simulink model "Control_Schematic_9"  (Simulink 8.3)
settings: Solver=FixedStepDiscrete  StartTime=0.0  StopTime=100  FixedStep=Ts  RelTol=1e-3
values from neighbouring files (symbols this model uses):
  b = 156    [StartUp_1.m]    (also in StartUp_11_Validation.m; StartUp_3.m; StartUp_4.m; StartUp_7.m)
  Eps = .1    (= 0.1)    [StartUp_9.m]
  K1 = PolyCon(1,2)    [StartUp_1.m]    (also in StartUp_4.m = 1; StartUp_7.m = 16; StartUp_8.m = 16; StartUp_9.m = 0.23)
  k2 = floor(rk(2,1))    [StartUp_9.m]
  K2 = 2    [StartUp_4.m]    (also in StartUp_7.m = 8; StartUp_8.m = 8; StartUp_9.m = 0.83)
  k3 = kk    [StartUp_9.m]
  K3 = 12000    [StartUp_9.m]
  ka = .5    (= 0.5)    [StartUp_9.m]
  Kn = .0019    (= 0.0019)    [StartUp_9.m]
  R = 50    [StartUp_1.m]    (also in StartUp_3.m; StartUp_4.m; StartUp_7.m; StartUp_8.m)
  Ts = 1/1000    (= 0.001)    [StartUp_1.m]    (also in StartUp_11_Validation.m = 0.01; StartUp_3.m; StartUp_4.m; StartUp_7.m)
  x_0 = 2500    [StartUp_9.m]
  y_0 = 2500    [StartUp_9.m]
undefined symbols (not defined in the file or in its folder): DiscIntNeverNeededParam
undefined symbols (not defined in the file): ADAMS_cwd, ADAMS_exec, ADAMS_host, ADAMS_init, ADAMS_inputs, ADAMS_outputs, ADAMS_prefix, ADAMS_static, ADAMS_sysdir
libraries: dspinverses x1, simulink x1
settings Model: Creator=baqumau  LastModifiedBy=baqumau
settings DataIOCC: SignalLoggingSaveFormat=Dataset
settings DebuggingCC: UnderspecifiedInitializationDetection=Simplified  StateNameClashWarn=none
settings GRTTargetCC: CombineOutputUpdateFcns=on  GRTInterface=off

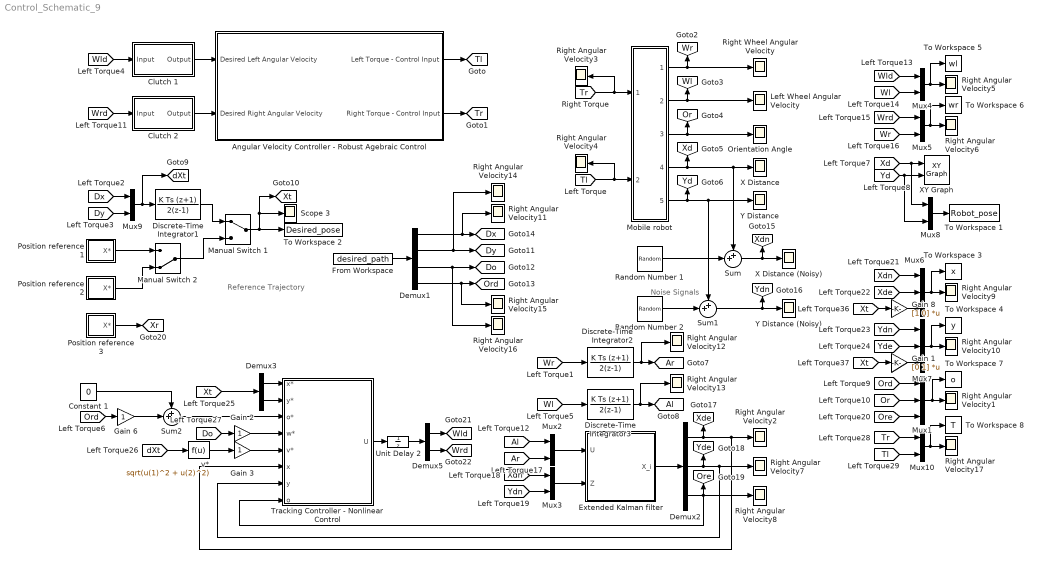
== system Control_Schematic_9 ==
  note: Noise Signals
  note: Reference Trajectory
  Angular Velocity Controller - Robust Agebraic Control : Subsystem
  Clutch 1 : Subsystem
  Clutch 2 : Subsystem
  Constant 1 : Constant  Value=0
  Demux1 : Demux
  Demux2 : Demux  Outputs=3
  Demux3 : Demux  Outputs=2
  Demux5 : Demux  Outputs=2
  Discrete-Time Integrator1 : DiscreteIntegrator  IntegratorMethod=Integration: Trapezoidal  gainval=1  InitialCondition=[x_0,y_0]'  SampleTime=Ts  ICPrevOutput=DiscIntNeverNeededParam  ICPrevScaledInput=DiscIntNeverNeededParam
  Discrete-Time Integrator2 : DiscreteIntegrator  IntegratorMethod=Integration: Trapezoidal  gainval=1  SampleTime=Ts  ICPrevOutput=DiscIntNeverNeededParam  ICPrevScaledInput=DiscIntNeverNeededParam
  Discrete-Time Integrator3 : DiscreteIntegrator  IntegratorMethod=Integration: Trapezoidal  gainval=1  SampleTime=Ts  ICPrevOutput=DiscIntNeverNeededParam  ICPrevScaledInput=DiscIntNeverNeededParam
  Extended Kalman filter : Subsystem
  From Workspace : FromWorkspace  VariableName=desired_path  SampleTime=Ts  OutputAfterFinalValue=Holding final value
  Gain 1 : Gain  Gain=[0 1]  Multiplication=Matrix(K*u)
  Gain 2 : Gain
  Gain 3 : Gain
  Gain 6 : Gain
  Gain 8 : Gain  Gain=[1 0]  Multiplication=Matrix(K*u)
  Left Wheel Angular Velocity : Scope
      settings: YMin=-1  YMax=1  SaveName=ScopeData2
  Manual Switch 1 : ManualSwitch
  Manual Switch 2 : ManualSwitch  CurrentSetting=0
  Mobile robot : Subsystem
  Mux1 : Mux  Inputs=3
  Mux{2..5,8..10} (7 alike) : Mux  Inputs=2
  Mux6 : Mux  Inputs=3
  Mux7 : Mux  Inputs=3
  Orientation Angle : Scope
      settings: YMin=-4  YMax=4
  Position reference 1 : Subsystem
  Position reference 2 : Subsystem
  Position reference 3 : Subsystem
  Random Number 1 : RandomNumber  Variance=.5  Seed=6
  Random Number 2 : RandomNumber  Variance=.5  Seed=8
  Right Angular Velocity{1..17} (17 alike) : Scope
      Right Angular Velocity1 settings: SaveName=ScopeData27
      Right Angular Velocity10 settings: YMin=0  YMax=5000  SaveName=ScopeData36
      Right Angular Velocity11 settings: YMin=0  YMax=4500  SaveName=ScopeData11
      Right Angular Velocity12 settings: YMin=-3  YMax=30  SaveName=ScopeData39
      Right Angular Velocity13 settings: YMin=-3  YMax=3  SaveName=ScopeData40
      Right Angular Velocity14 settings: TimeRange=500  YMin=0  YMax=4500  SaveName=ScopeData13
      Right Angular Velocity15 settings: YMin=-3.141592653589793  YMax=3.141592653589793  SaveName=ScopeData15
      Right Angular Velocity16 settings: YMin=0  YMax=4500  SaveName=ScopeData16
      Right Angular Velocity17 settings: YMax=25  SaveName=ScopeData5
      Right Angular Velocity2 settings: YMin=2400  YMax=2600  SaveName=ScopeData24
      Right Angular Velocity3 settings: YMin=-25  YMax=25  SaveName=ScopeData7
      Right Angular Velocity4 settings: YMin=-25  YMax=25  SaveName=ScopeData8
      Right Angular Velocity5 settings: YMax=25  SaveName=ScopeData9
      Right Angular Velocity6 settings: TimeRange=388.54  YMin=-3  YMax=25  SaveName=ScopeData10
      Right Angular Velocity7 settings: YMin=0  YMax=5000  SaveName=ScopeData25
      Right Angular Velocity8 settings: YMin=-3.141592653589793  YMax=3.141592653589793  SaveName=ScopeData26
      Right Angular Velocity9 settings: YMin=0  YMax=5000  SaveName=ScopeData35
  Right Wheel Angular Velocity : Scope
      settings: YMin=-1  YMax=1  SaveName=ScopeData3
  Scope 3 : Scope
      settings: YMin=100  YMax=5000  SaveName=ScopeData37
  Sum : Sum  Inputs=++|
  Sum1 : Sum  Inputs=++|
  Sum2 : Sum  Inputs=++|
  To Workspace 1 : ToWorkspace  VariableName=Robot_pose  SaveFormat=Structure With Time  SampleTime=-1
  To Workspace 2 : ToWorkspace  VariableName=Desired_pose  SaveFormat=Structure With Time  SampleTime=-1
  To Workspace 3 : ToWorkspace  VariableName=x  SaveFormat=Structure With Time  SampleTime=-1
  To Workspace 4 : ToWorkspace  VariableName=y  SaveFormat=Structure With Time  SampleTime=-1
  To Workspace 5 : ToWorkspace  VariableName=wl  SaveFormat=Structure With Time  SampleTime=-1
  To Workspace 6 : ToWorkspace  VariableName=wr  SaveFormat=Structure With Time  SampleTime=-1
  To Workspace 7 : ToWorkspace  VariableName=o  SaveFormat=Structure With Time  SampleTime=-1
  To Workspace 8 : ToWorkspace  VariableName=T  SaveFormat=Structure With Time  SampleTime=-1
  Tracking Controller - Nonlinear Control : Subsystem
  Unit Delay 2 : UnitDelay  SampleTime=-1
  X Distance : Scope
      settings: YMin=0  YMax=5000  SaveName=ScopeData4
  X Distance (Noisy) : Scope
      settings: YMin=0  YMax=2600  SaveName=ScopeData19
  XY Graph : simulink/Sinks/XY Graph  xmin=0  xmax=5000  ymin=0  ymax=5000  st=Ts
  Y Distance : Scope
      settings: YMin=0  YMax=5000
  Y Distance (Noisy) : Scope
      settings: YMin=0  YMax=2600  SaveName=ScopeData21
  v* : Fcn  Expr=sqrt(u(1)^2 + u(2)^2)
  tag scope: Al=global, Ar=global, Do=global, Dx=global, Dy=global, Or=global, Ord=global, Ore=global, Tl=global, Tr=global, Wl=global, Wld=global, Wr=global, Wrd=global, Xd=global, Xde=global, Xdn=global, Xr=global, Xt=global, Yd=global, Yde=global, Ydn=global, dXt=global
  wires:
  Mobile robot/1(Wrw) -> Right Wheel Angular Velocity/1, [Wr]
  Mobile robot/2(Wlw) -> Left Wheel Angular Velocity/1, [Wl]
  Mobile robot/3(Alpha) -> Orientation Angle/1, [Or]
  Mobile robot/4(X_Dist) -> Sum/1, X Distance/1, [Xd]
  Mobile robot/5(Y_Dist) -> Y Distance/1, Sum1/1, [Yd]
  [Tr] -> Mobile robot/1(Trw), Right Angular Velocity3/1
  [Tl] -> Mobile robot/2(Tlw), Right Angular Velocity4/1
  [Wld] -> Mux4/1
  [Wl] -> Mux4/2
  Mux4/1 -> To Workspace 5/1, Right Angular Velocity5/1
  [Wrd] -> Mux5/1
  [Wr] -> Mux5/2
  Mux5/1 -> To Workspace 6/1, Right Angular Velocity6/1
  [Xd] -> Mux8/1, XY Graph/1
  [Yd] -> Mux8/2, XY Graph/2
  [Ord] -> Mux1/1
  [Or] -> Mux1/2
  Mux1/1 -> To Workspace 7/1, Right Angular Velocity1/1
  Random Number 1/1 -> Sum/2
  Sum1/1 -> Y Distance (Noisy)/1, [Ydn]
  Sum/1 -> [Xdn], X Distance (Noisy)/1
  [Ar] -> Mux2/2
  [Al] -> Mux2/1
  [Ydn] -> Mux3/2
  [Xdn] -> Mux3/1
  Mux2/1 -> Extended Kalman filter/1(U)
  Mux3/1 -> Extended Kalman filter/2(Z)
  Demux2/2 -> [Yde], Tracking Controller - Nonlinear Control/7(y), Right Angular Velocity7/1
  Demux2/3 -> Tracking Controller - Nonlinear Control/8(o), [Ore], Right Angular Velocity8/1
  Demux2/1 -> [Xde], Tracking Controller - Nonlinear Control/6(x), Right Angular Velocity2/1
  [Ore] -> Mux1/3
  [Xdn] -> Mux6/1
  Mux6/1 -> To Workspace 3/1, Right Angular Velocity9/1
  [Xde] -> Mux6/2
  [Ydn] -> Mux7/1
  Mux7/1 -> To Workspace 4/1, Right Angular Velocity10/1
  [Yde] -> Mux7/2
  Mux8/1 -> To Workspace 1/1
  [Xt] -> Gain 8/1
  Gain 8/1 -> Mux6/3
  [Xt] -> Gain 1/1
  Gain 1/1 -> Mux7/3
  Manual Switch 1/1 -> [Xt], Scope 3/1, To Workspace 2/1
  Demux1/1 -> Right Angular Velocity11/1, [Dx]
  Demux1/2 -> Right Angular Velocity14/1, [Dy]
  Demux1/3 -> Right Angular Velocity16/1, [Do]
  Demux1/4 -> Right Angular Velocity15/1, [Ord]
  From Workspace/1 -> Demux1/1
  [Dx] -> Mux9/1
  [Dy] -> Mux9/2
  Mux9/1 -> [dXt], Discrete-Time Integrator1/1
  Discrete-Time Integrator1/1 -> Manual Switch 1/1
  Position reference 1/1(X*) -> Manual Switch 2/1
  Manual Switch 2/1 -> Manual Switch 1/2
  Position reference 2/1(X*) -> Manual Switch 2/2
  Position reference 3/1(X*) -> [Xr]
  Demux5/2 -> [Wrd]
  Demux5/1 -> [Wld]
  Discrete-Time Integrator2/1 -> Right Angular Velocity12/1, [Ar]
  [Wr] -> Discrete-Time Integrator2/1
  Discrete-Time Integrator3/1 -> Right Angular Velocity13/1, [Al]
  [Wl] -> Discrete-Time Integrator3/1
  Tracking Controller - Nonlinear Control/1(U) -> Unit Delay 2/1
  Demux3/1 -> Tracking Controller - Nonlinear Control/1(x*)
  Demux3/2 -> Tracking Controller - Nonlinear Control/2(y*)
  [Xt] -> Demux3/1
  [Wld] -> Clutch 1/1(Input)
  [Wrd] -> Clutch 2/1(Input)
  [Do] -> Gain 2/1
  v*/1 -> Gain 3/1
  [dXt] -> v*/1
  Clutch 1/1(Output) -> Angular Velocity Controller - Robust Agebraic Control/1(Desired Left Angular Velocity)
  Clutch 2/1(Output) -> Angular Velocity Controller - Robust Agebraic Control/2(Desired Right Angular Velocity)
  [Ord] -> Gain 6/1
  Extended Kalman filter/1(X_i) -> Demux2/1
  Unit Delay 2/1 -> Demux5/1
  Angular Velocity Controller - Robust Agebraic Control/2(Right Torque - Control Input) -> [Tr]
  Angular Velocity Controller - Robust Agebraic Control/1(Left Torque - Control Input) -> [Tl]
  Random Number 2/1 -> Sum1/2
  [Tr] -> Mux10/1
  [Tl] -> Mux10/2
  Mux10/1 -> Right Angular Velocity17/1, To Workspace 8/1
  Gain 2/1 -> Tracking Controller - Nonlinear Control/4(w*)
  Gain 3/1 -> Tracking Controller - Nonlinear Control/5(v*)
  Sum2/1 -> Tracking Controller - Nonlinear Control/3(o*)
  Gain 6/1 -> Sum2/2
  Constant 1/1 -> Sum2/1

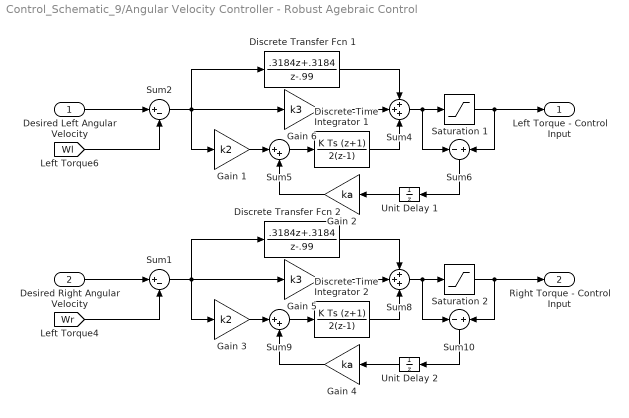
== system Control_Schematic_9/Angular Velocity Controller - Robust Agebraic Control ==
  Desired Left Angular Velocity : Inport
  Desired Right Angular Velocity : Inport  Port=2
  Discrete Transfer Fcn 1 : DiscreteTransferFcn  Numerator=[.3184 .3184]  Denominator=[1 -.99]  SampleTime=Ts
  Discrete Transfer Fcn 2 : DiscreteTransferFcn  Numerator=[.3184 .3184]  Denominator=[1 -.99]  SampleTime=Ts
  Discrete-Time Integrator 1 : DiscreteIntegrator  IntegratorMethod=Integration: Trapezoidal  SampleTime=Ts  ICPrevOutput=DiscIntNeverNeededParam  ICPrevScaledInput=DiscIntNeverNeededParam
  Discrete-Time Integrator 2 : DiscreteIntegrator  IntegratorMethod=Integration: Trapezoidal  SampleTime=Ts  ICPrevOutput=DiscIntNeverNeededParam  ICPrevScaledInput=DiscIntNeverNeededParam
  Gain 1 : Gain  Gain=k2
  Gain 2 : Gain  Gain=ka
  Gain 3 : Gain  Gain=k2
  Gain 4 : Gain  Gain=ka
  Gain 5 : Gain  Gain=k3
  Gain 6 : Gain  Gain=k3
  Saturation 1 : Saturate  UpperLimit=15  LowerLimit=-15
  Saturation 2 : Saturate  UpperLimit=15  LowerLimit=-15
  Sum1 : Sum  Inputs=|+-
  Sum10 : Sum  Inputs=-+
  Sum2 : Sum  Inputs=|+-
  Sum4 : Sum  Inputs=+++
  Sum5 : Sum  Inputs=|++
  Sum6 : Sum  Inputs=-+
  Sum8 : Sum  Inputs=+++
  Sum9 : Sum  Inputs=|++
  Unit Delay 1 : UnitDelay  SampleTime=-1
  Unit Delay 2 : UnitDelay  SampleTime=-1
  Left Torque - Control Input : Outport
  Right Torque - Control Input : Outport  Port=2
  wires:
  Desired Right Angular Velocity/1 -> Sum1/1
  Desired Left Angular Velocity/1 -> Sum2/1
  Saturation 1/1 -> Left Torque - Control Input/1, Sum6/2
  Sum4/1 -> Sum6/1, Saturation 1/1
  Sum2/1 -> Discrete Transfer Fcn 1/1, Gain 1/1, Gain 6/1
  Discrete Transfer Fcn 1/1 -> Sum4/1
  Gain 1/1 -> Sum5/1
  Sum5/1 -> Discrete-Time Integrator 1/1
  Discrete-Time Integrator 1/1 -> Sum4/3
  Sum6/1 -> Unit Delay 1/1
  Gain 2/1 -> Sum5/2
  Saturation 2/1 -> Right Torque - Control Input/1, Sum10/2
  Sum8/1 -> Saturation 2/1, Sum10/1
  Sum1/1 -> Discrete Transfer Fcn 2/1, Gain 5/1, Gain 3/1
  Discrete Transfer Fcn 2/1 -> Sum8/1
  Gain 3/1 -> Sum9/1
  Sum9/1 -> Discrete-Time Integrator 2/1
  Discrete-Time Integrator 2/1 -> Sum8/3
  Sum10/1 -> Unit Delay 2/1
  Gain 4/1 -> Sum9/2
  Unit Delay 1/1 -> Gain 2/1
  Unit Delay 2/1 -> Gain 4/1
  Gain 5/1 -> Sum8/2
  Gain 6/1 -> Sum4/2
  [Wl] -> Sum2/2
  [Wr] -> Sum1/2

== system Control_Schematic_9/Clutch 1 ==
  Input : Inport
  Constant1 : Constant  Value=2
  Digital Clock : DigitalClock  SampleTime=Ts
  Gain 1 : Gain  Gain=.5
  Product : Product
  Rear Wheel Angular Speed5 : Scope
      settings: YMin=0  YMax=2  SaveName=ScopeData5
  Sine Wave1 : Sin  Bias=1  Frequency=(pi/5)  Phase=-pi/2  SampleTime=Ts
  Switch : Switch  Threshold=5
  Output : Outport
  wires:
  Constant1/1 -> Switch/1
  Digital Clock/1 -> Switch/2
  Switch/1 -> Gain 1/1
  Input/1 -> Product/2
  Product/1 -> Output/1
  Sine Wave1/1 -> Switch/3
  Gain 1/1 -> Rear Wheel Angular Speed5/1, Product/1

== system Control_Schematic_9/Clutch 2 ==
  Input : Inport
  Constant1 : Constant  Value=2
  Digital Clock : DigitalClock  SampleTime=Ts
  Gain 1 : Gain  Gain=.5
  Product : Product
  Rear Wheel Angular Speed5 : Scope
      settings: YMin=0  YMax=2  SaveName=ScopeData5
  Sine Wave1 : Sin  Bias=1  Frequency=(pi/5)  Phase=-pi/2  SampleTime=Ts
  Switch : Switch  Threshold=5
  Output : Outport
  wires:
  Gain 1/1 -> Product/1, Rear Wheel Angular Speed5/1
  Sine Wave1/1 -> Switch/3
  Product/1 -> Output/1
  Input/1 -> Product/2
  Switch/1 -> Gain 1/1
  Digital Clock/1 -> Switch/2
  Constant1/1 -> Switch/1

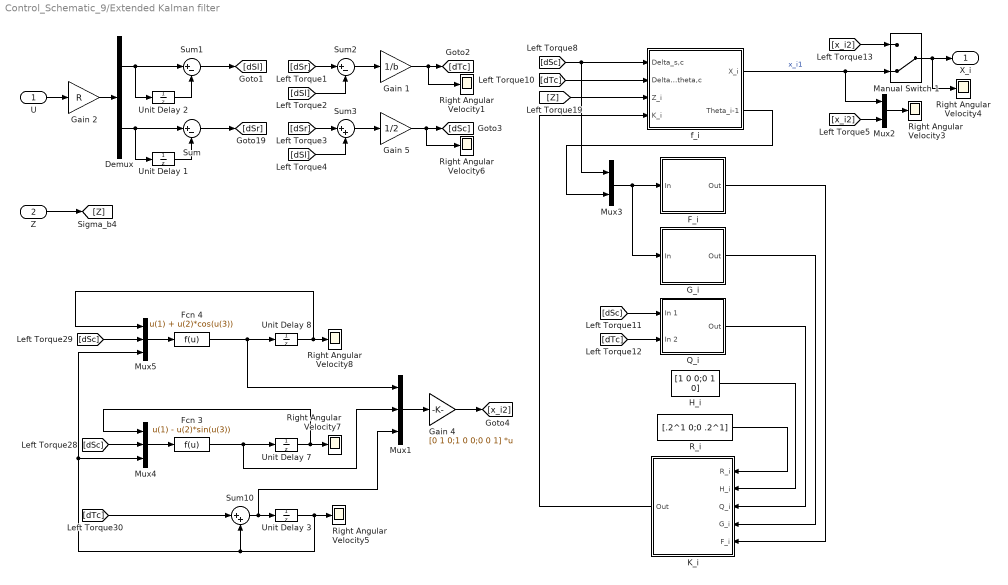
== system Control_Schematic_9/Extended Kalman filter ==
  U : Inport
  Z : Inport  Port=2
  Demux : Demux  Outputs=2
  F_i : Subsystem
  Fcn 3 : Fcn  Expr=u(1) - u(2)*sin(u(3))
  Fcn 4 : Fcn  Expr=u(1) + u(2)*cos(u(3))
  G_i : Subsystem
  Gain 1 : Gain  Gain=1/b
  Gain 2 : Gain  Gain=R
  Gain 4 : Gain  Gain=[0 1 0;1 0 0;0 0 1]  Multiplication=Matrix(K*u)
  Gain 5 : Gain  Gain=1/2
  H_i : Constant  Value=[1 0 0;0 1 0]
  K_i : Subsystem
  Manual Switch 1 : ManualSwitch  CurrentSetting=0
  Mux1 : Mux  Inputs=3
  Mux2 : Mux  Inputs=2
  Mux3 : Mux  Inputs=2
  Mux4 : Mux  Inputs=3
  Mux5 : Mux  Inputs=3
  Q_i : Subsystem
  R_i : Constant  Value=[.2^1 0;0 .2^1]
  Right Angular Velocity{1,3..8} (7 alike) : Scope
      Right Angular Velocity1 settings: YMin=-1  YMax=1  SaveName=ScopeData23
      Right Angular Velocity3 settings: YMin=-1  YMax=2  SaveName=ScopeData29
      Right Angular Velocity4 settings: YMin=-1  YMax=1  SaveName=ScopeData31
      Right Angular Velocity5 settings: YMin=-1  YMax=3  SaveName=ScopeData32
      Right Angular Velocity6 settings: YMin=-1  YMax=1  SaveName=ScopeData22
      Right Angular Velocity7 settings: YMin=2490  YMax=2510  SaveName=ScopeData33
      Right Angular Velocity8 settings: YMin=100  YMax=500  SaveName=ScopeData34
  Sum : Sum  Inputs=|+-
  Sum1 : Sum  Inputs=|+-
  Sum10 : Sum  Inputs=|++
  Sum2 : Sum  Inputs=|+-
  Sum3 : Sum  Inputs=|++
  Unit Delay 1 : UnitDelay  SampleTime=-1
  Unit Delay 2 : UnitDelay  SampleTime=-1
  Unit Delay 3 : UnitDelay  SampleTime=-1
  Unit Delay 7 : UnitDelay  InitialCondition=2500  SampleTime=-1
  Unit Delay 8 : UnitDelay  InitialCondition=200  SampleTime=-1
  f_i : Subsystem
  X_i : Outport
  wires:
  U/1 -> Gain 2/1
  Demux/2 -> Unit Delay 1/1, Sum/1
  Unit Delay 1/1 -> Sum/2
  Sum/1 -> [dSr]
  Demux/1 -> Sum1/1, Unit Delay 2/1
  Unit Delay 2/1 -> Sum1/2
  Sum1/1 -> [dSl]
  [dSr] -> Sum2/1
  [dSl] -> Sum2/2
  Sum2/1 -> Gain 1/1
  Gain 1/1 -> Right Angular Velocity1/1, [dTc]
  [dSr] -> Sum3/1
  [dSl] -> Sum3/2
  Sum3/1 -> Gain 5/1
  Gain 5/1 -> Right Angular Velocity6/1, [dSc]
  [dSc] -> Mux3/1, f_i/1(Delta_s,c)
  Mux3/1 -> G_i/1(In), F_i/1(In)
  Sum10/1 -> Mux1/3, Unit Delay 3/1
  Unit Delay 3/1 -> Right Angular Velocity5/1, Mux5/3, Mux4/3, Sum10/2
  Unit Delay 7/1 -> Mux4/1, Right Angular Velocity7/1
  Fcn 3/1 -> Mux1/2, Unit Delay 7/1
  [dSc] -> Mux4/2
  Mux4/1 -> Fcn 3/1
  Fcn 4/1 -> Mux1/1, Unit Delay 8/1
  Mux5/1 -> Fcn 4/1
  Unit Delay 8/1 -> Mux5/1, Right Angular Velocity8/1
  [dSc] -> Mux5/2
  Gain 2/1 -> Demux/1
  Z/1 -> [Z]
  [Z] -> f_i/3(Z_i)
  [dTc] -> f_i/2(Delta_theta,c)
  [dSc] -> Q_i/1(In 1)
  [dTc] -> Q_i/2(In 2)
  Mux1/1 -> Gain 4/1
  Gain 4/1 -> [x_i2]
  Manual Switch 1/1 -> Right Angular Velocity4/1, X_i/1
  [x_i2] -> Manual Switch 1/1
  f_i/1(X_i) -> Mux2/1, Manual Switch 1/2  "x_i1"
  [x_i2] -> Mux2/2
  Mux2/1 -> Right Angular Velocity3/1
  [dTc] -> Sum10/1
  K_i/1(Out) -> f_i/4(K_i)
  f_i/2(Theta_i-1) -> Mux3/2
  F_i/1(Out) -> K_i/5(F_i)
  G_i/1(Out) -> K_i/4(G_i)
  Q_i/1(Out) -> K_i/3(Q_i)
  H_i/1 -> K_i/2(H_i)
  R_i/1 -> K_i/1(R_i)

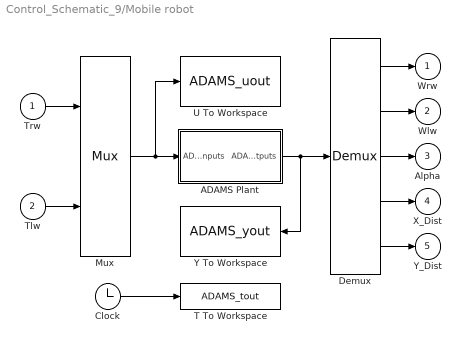
== system Control_Schematic_9/Mobile robot ==
  Trw : Inport
  Tlw : Inport  Port=2
  ADAMS Plant : Subsystem  LoadFcn=|  InitFcn=clear mex  mask(Adams Plant){exevie=ADAMS_sysdir, nam_in=ADAMS_inputs, namout=ADAMS_outputs, nampre=ADAMS_prefix, outfil=ADAMS_prefix, exesol=ADAMS_exec, stat=ADAMS_static, inicmd=[ADAMS_init], exetyp=C++, comtyp=PIPE(DDE), workdir=ADAMS_cwd, ada_host=ADAMS_host, modani=batch, modsim=discrete, dft=no, simulink_lead_cosim=yes, pin_interp_order=0, pout_extrap_order=0, pin_extrap_order=0, pout_interp_order=0, dt_out=Ts, o_rate=1, more=off}
      | %check based on dialog box setting for when setting by popup menu                                             
      | if exist('ADAMS_solver_type')                                                                                 
      |   if strcmp(ADAMS_solver_type,'C++')                                                                          
      |     set_param(gcb,'exetyp','C++');                                                                            
      |   else                                                                                                        
      |     set_param(gcb,'exetyp','Fortran');                                                                        
      |   end                                                                                                         
      | else                                                                                                          
      |   set_param(gcb,'exetyp','C++');                                                                              
      | end                                                                                                           
      | %set the mode if using acar_solver                                                                            
      | %REQUIRED HERE BECAUSE BELOW CAUSES MDLTERMINATE TO BE CALLED 2 TIMES IN MIDDLE OF SIMULATION WHEN SET IN MASK
      |                                                                                                               
      | %enable the direct feedthrough, sim mode, anim mode parameters by default                                     
      |                                                                                                               
      | if exist('set_some_params_states')                                                                            
      |                                                                                                               
      |   set_some_params_states({'dft','modsim','modani'},{'on','on','on'},'MaskEnables',gcb)                        
      |   %turn on direct feedthrough option                                                                          
      |   set_some_params_states({'dft'},{'on'},'MaskVisibilities',gcb)                                               
      |                                                                                                               
      |  end                                                                                                          
      |                                                                                                               
      |                                                                                                               
      | if exist('ADAMS_exec')                                                                                        
      |   if and(strcmp(get_param(gcb,'exesol'),'ADAMS_exec'),strcmp(ADAMS_exec,'acar_solver'))                       
      |     %set the sim mode to discrete -- only supported mode                                                      
      |     set_param(gcb,'modsim','discrete')                                                                        
      |      %turn off direct feedthrough option                                                                      
      |      set_some_params_states({'dft'},{'off'},'MaskVisibilities',gcb)                                           
      |     %set the animation mode to batch -- only supported mode                                                   
      |     set_param(gcb,'modani','batch')                                                                           
      |     %disable the direct feedthrough, sim mode, anim mode parameters                                           
      |     set_some_params_states({'modsim','modani'},{'off','off'},'MaskEnables',gcb)                               
      |   end                                                                                                         
      | end
      mask prompts: exevie "Adams install directory"; nam_in "Adams/View input names"; namout "Adams/View output names"; nampre "Adams model file prefix"; outfil "Output files prefix (opt.: if blank - no output)"; exesol "User executable (opt.: if blank - use standard)"; stat "Initial static simulation flag"; inicmd "Initialization commands"; exetyp "Adams/Solver type"; comtyp "Interprocess option"; workdir "Adams working directory"; ada_host "Adams host"; modani "Animation mode"; modsim "Simulation mode"; dft "Direct feedthrough"; simulink_lead_cosim "Discrete Computational Order - Simulink Leads Adams"; pin_interp_order "Plant input interpolation order"; pout_extrap_order "Plant output extrapolation order"; pin_extrap_order "Plant input extrapolation order"; pout_interp_order "Plant output interpolation order"; dt_out "Communication interval"; o_rate "Number of communications per output step"; more "More parameters"
      mask help: Simulate any Adams plant model either in Adams/Solver form (.adm file) or in Adams/View form (.cmd file)
      settings: OpenFcn=|
      | open_system(gcb,'mask')
      | if not(exist('set_some_params_states'))
      | 
      | warning('The script "set_some_params_states.m" cannot be found in the MATLAB PATH.  Cannot update the ADAMS Plant S-Function parameters.')
      | 
      | warning('Recommended action(optional):  run the Adams/Controls .m file first to help choose the correct settings in the Adams S-Function block.')
      | 
      | end
      mask Help:
      | <html>
      | This S-Function represents the non-linear Adams Plant with the inputs sent to the Adams model <br>
      |  and the outputs generated by the Adams model.  See the Adams/Controls documentation for more <br>
      | information.  This plant uses the following variables:<br>
      | <br>
      | <b>ADAMS_sysdir  :</b> Adams installation directory<br>
      | <b>ADAMS_inputs  :</b> Input variables View names vector<br>
      | <b>ADAMS_outputs :</b> Outputs variables View names vector<br>
      | <b>ADAMS_prefix  : </b>ADAMS model files prefix (.adm, .cmd); also doubles as output files prefix<br>
      | <b>ADAMS_exec :</b> Adams/Solver user library or keyword (e.g., acar_solver)<br>
      | <b>ADAMS_static :</b> yes|no - initial static before Co-simulation(discrete)/Function Evaluation(continuous)<br>
      | <b>ADAMS_init :</b>Initialization commands (i.e., Adams/View or Solver commands, depending on setting for Animation mode)<br>
      | <b>ADAMS_cwd : </b> Current working directory (for TCP/IP)<br>
      | <b>ADAMS_host : </b>Name of Adams server host (for TCP/IP)<br>
      | <b>ADAMS_mode :</b> Linear or non-linear (i.e., co-sim, function eval)<br>
      | <b>ADAMS_solver_type :</b>Fortran or C++ (used to set popup menu when first loaded) <br>
      | 
      | 
      | <br>
      | The following settings can be chosen:<br>
      | <br>
      | <b>Adams/Solver type:</b>  Fortran or C++ (will also set ADAMS_solver_type)<br>
      | <b>Interprocess option:</b> Pipe(DDE) or TCP/IP; TCP/IP can allow different machines run Adams and MATLAB<br>
      | <b>Animation mode:</b> batch (Solver, uses .adm) or interactive (View, uses .cmd)<br>
      | <b>Simulation mode:</b> discrete (Co-simulation) or continuous (Function Evaluation)<br>
      | <b>Discrete Computational Order - Simulink Lead Adams:</b> for discrete mode, chooses if Simulink leads the integration (yes) or lags (no);<br> if set to "no", can remove algebraic loop<br>
      | <b>Plant input interpolation order:</b> 0 = zero-order hold; 1 = linear (discrete mode only, where Simulink leads)<br>
      | <b>Plant output extrapolation order:</b> 0 = zero-order hold;1 = linear(discrete mode only, where Simulink leads)<br>
      | <b>Plant input extrapolation order:</b> 0 = zero-order hold; 1 = linear (discrete mode only, where Adams leads)<br>
      | <b>Plant output interpolation order:</b> 0 = zero-order hold;1 = linear(discrete mode only, where Adams leads)<br>
      | <b>Direct feedthrough:</b> yes|no - yes = Input directly effect output(continuous mode-only)<br>
      | <b>Communication interval:</b> Time step at which Co-simulation exchange information (e.g.,0.005); also controls <br>output for continuous mode (Function Evaluation)<br>
      | <b>Number of communications per output step: </b>Sets Adams output rate (.res, .req, .gra) integer value (default: 1)<br>
      | </html>
      mask Callback exesol:
      | if exist('set_some_params_states')
      | %enable the direct feedthrough, sim mode, anim mode parameters
      | set_some_params_states({'dft','modsim','modani'},{'on','on','on'},'MaskEnables',gcb)
      | %turn on direct feedthrough option
      | set_some_params_states({'dft'},{'on'},'MaskVisibilities',gcb)
      | end
      | 
      | if exist('ADAMS_exec')
      |   if and(strcmp(get_param(gcb,'exesol'),'ADAMS_exec'),strcmp(ADAMS_exec,'acar_solver'))
      |     %set the sim mode to discrete -- only supported mode
      |     %REMOVED:  BELOW CAUSES MDLTERMINATE TO BE CALLED 2 TIMES IN MIDDLE OF SIMULATION
      |     %Now in LoadFcn callback
      |     %set_param(gcb,'modsim','discrete')
      |      %turn off direct feedthrough option
      |     set_some_params_states({'dft'},{'off'},'MaskVisibilities',gcb)
      |     %set the animation mode to batch -- only supported mode
      |     %REMOVED:  BELOW CAUSES MDLTERMINATE TO BE CALLED 2 TIMES IN MIDDLE OF SIMULATION
      |     %Now in LoadFcn callback
      |     %set_param(gcb,'modani','batch')
      |     %disable the direct feedthrough, sim mode, anim mode parameters
      |     set_some_params_states({'modsim','modani'},{'off','off'},'MaskEnables',gcb)
      |   end
      | end
      mask TypeOptions exetyp: Fortran | C++
      mask Callback exetyp:
      | if strcmp(get_param(gcb,'exetyp'),'C++')
      |     ADAMS_solver_type='C++';
      | else
      |     ADAMS_solver_type='Fortran';
      | end
      mask TypeOptions comtyp: PIPE(DDE) | TCP/IP
      mask Callback comtyp:
      | if exist('set_some_params_states')
      | if strcmp(get_param(gcb,'comtyp'),'PIPE(DDE)')
      |     %turn off cwd, host options
      |     set_some_params_states({'ada_host','workdir'},{'off','off'},'MaskVisibilities',gcb)
      | else%if strcmp(get_param(gcb,'modsim'),'TCP/IP')
      |     %turn on cwd, host options
      |     set_some_params_states({'ada_host','workdir'},{'on','on'},'MaskVisibilities',gcb)
      | end
      | end
      mask TypeOptions modani: batch | interactive
      mask TypeOptions modsim: discrete | continuous
      mask Callback modsim:
      | if exist('set_some_params_states')
      | if strcmp(get_param(gcb,'modsim'),'discrete')
      |      %turn off direct feedthrough option
      |     set_some_params_states({'dft'},{'off'},'MaskVisibilities',gcb)
      |     %turn on discrete co-sim type if want to see more
      |     if strcmp(get_param(gcb,'more'),'on')
      |         set_some_params_states({'simulink_lead_cosim'},{'on'},'MaskVisibilities',gcb)
      |     end
      |     if strcmp(get_param(gcb,'simulink_lead_cosim'),'yes')
      |         %turn on interpolation/extrapolation options
      |         set_some_params_states({'pin_interp_order','pout_extrap_order',},{'on','on'},'MaskVisibilities',gcb)
      |     else
      |         set_some_params_states({'pin_extrap_order','pout_interp_order'},{'on','on'},'MaskVisibilities',gcb)
      |     end
      | else%if strcmp(get_param(gcb,'modsim'),'continuous')
      |      %turn off direct feedthrough option
      |     set_some_params_states({'dft'},{'on'},'MaskVisibilities',gcb)
      |     %turn off interpolation/extrapolation options
      |     set_some_params_states({'pin_interp_order','pout_extrap_order','pin_extrap_order','pout_interp_order','simulink_lead_cosim'},{'off','off','off','off','off'},'MaskVisibilities',gcb)
      | end
      | end
      mask TypeOptions dft: no | yes
      mask TypeOptions simulink_lead_cosim: yes | no
      mask Callback simulink_lead_cosim:
      | if exist('set_some_params_states')
      | if (strcmp(get_param(gcb,'simulink_lead_cosim'),'yes') && strcmp(get_param(gcb,'modsim'),'discrete'))
      |      %turn off unused interpolate/extrapolate options
      |     set_some_params_states({'pin_extrap_order','pout_interp_order'},{'off','off'},'MaskVisibilities',gcb)
      |     %turn on used interpolate/extrapolate options
      |     set_some_params_states({'pin_interp_order','pout_extrap_order'},{'on','on'},'MaskVisibilities',gcb)
      | elseif (strcmp(get_param(gcb,'simulink_lead_cosim'),'no') && strcmp(get_param(gcb,'modsim'),'discrete'))
      |     %turn on used interpolate/extrapolate options
      |     set_some_params_states({'pin_extrap_order','pout_interp_order'},{'on','on'},'MaskVisibilities',gcb)
      |      %turn off unused interpolate/extrapolate options
      |     set_some_params_states({'pin_interp_order','pout_extrap_order'},{'off','off'},'MaskVisibilities',gcb)
      | end
      | end
      mask TypeOptions pin_interp_order: 0 | 1
      mask TypeOptions pout_extrap_order: 0 | 1
      mask TypeOptions pin_extrap_order: 0 | 1
      mask TypeOptions pout_interp_order: 0 | 1
      mask Callback more:
      | if exist('set_some_params_states')
      | if (strcmp(get_param(gcb,'more'),'on'))
      |      %turn on infrequently used options
      |     set_some_params_states({'exevie','nam_in','namout','exesol','stat','inicmd'},{'on','on','on','on','on','on'},'MaskVisibilities',gcb)
      |     if strcmp(get_param(gcb,'modsim'),'discrete')
      |         set_some_params_states({'simulink_lead_cosim'},{'on'},'MaskVisibilities',gcb)
      |     end
      | elseif (strcmp(get_param(gcb,'more'),'off'))
      |     %turn off infrequently used options
      |     set_some_params_states({'exevie','nam_in','namout','exesol','stat','inicmd'},{'off','off','off','off','off','off'},'MaskVisibilities',gcb)
      |     if strcmp(get_param(gcb,'modsim'),'discrete')
      |         set_some_params_states({'simulink_lead_cosim'},{'off'},'MaskVisibilities',gcb)
      |     end
      | end
      | end
      mask Display: disp( 'MSC Software' )
  Clock : Clock
  Demux : Demux  Outputs=5
  Mux : Mux  Inputs=2
  T To Workspace : ToWorkspace  VariableName=ADAMS_tout
      settings: MaxDataPoints=100000
  U To Workspace : ToWorkspace  VariableName=ADAMS_uout
      settings: MaxDataPoints=100000
  Y To Workspace : ToWorkspace  VariableName=ADAMS_yout
      settings: MaxDataPoints=100000
  Wrw : Outport
  Wlw : Outport  Port=2
  Alpha : Outport  Port=3
  X_Dist : Outport  Port=4
  Y_Dist : Outport  Port=5
  wires:
  Tlw/1 -> Mux/2
  Trw/1 -> Mux/1
  Demux/5 -> Y_Dist/1
  Demux/4 -> X_Dist/1
  Demux/3 -> Alpha/1
  Demux/2 -> Wlw/1
  Demux/1 -> Wrw/1
  ADAMS Plant/1(ADAMS outputs) -> Y To Workspace/1, Demux/1
  Mux/1 -> U To Workspace/1, ADAMS Plant/1(ADAMS inputs)
  Clock/1 -> T To Workspace/1

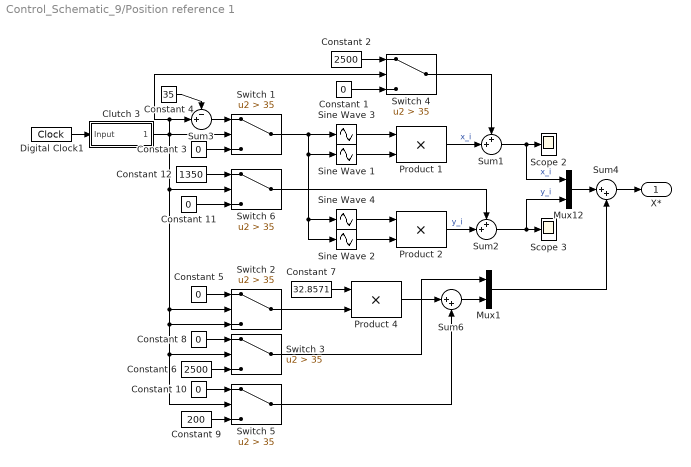
== system Control_Schematic_9/Position reference 1 ==
  Clutch 3 : Subsystem
  Constant {1,3,5,8,10..11} (6 alike) : Constant  Value=0
  Constant 12 : Constant  Value=1350
  Constant 2 : Constant  Value=2500
  Constant 4 : Constant  Value=35
  Constant 6 : Constant  Value=2500
  Constant 7 : Constant  Value=32.8571
  Constant 9 : Constant  Value=200
  Digital Clock1 : DigitalClock  SampleTime=Ts
  Mux1 : Mux  Inputs=2
  Mux12 : Mux  Inputs=2
  Product 1 : Product
  Product 2 : Product
  Product 4 : Product
  Scope 2 : Scope
      settings: YMin=-10  YMax=10
  Scope 3 : Scope
      settings: YMin=-10  YMax=10
  Sine Wave 1 : Sin  TimeSource=Use external signal  Amplitude=600  Frequency=2*pi/120  SampleTime=0
  Sine Wave 2 : Sin  TimeSource=Use external signal  Amplitude=600  Frequency=2*pi/120  SampleTime=0
  Sine Wave 3 : Sin  TimeSource=Use external signal  Frequency=2*pi/90  SampleTime=0
  Sine Wave 4 : Sin  TimeSource=Use external signal  Frequency=2*pi/90  Phase=pi/2  SampleTime=0
  Sum1 : Sum  Inputs=++|
  Sum2 : Sum  Inputs=++|
  Sum3 : Sum  Inputs=-+|
  Sum4 : Sum  Inputs=|++
  Sum6 : Sum  Inputs=|++
  Switch {1..6} (6 alike) : Switch  Criteria=u2 > Threshold  Threshold=35
  X* : Outport
  wires:
  Sine Wave 3/1 -> Product 1/1
  Sine Wave 4/1 -> Product 2/1
  Sine Wave 1/1 -> Product 1/2
  Sine Wave 2/1 -> Product 2/2
  Product 1/1 -> Sum1/2  "x_i"
  Sum2/1 -> Mux12/2, Scope 3/1  "y_i"
  Sum1/1 -> Mux12/1, Scope 2/1  "x_i"
  Product 2/1 -> Sum2/2  "y_i"
  Digital Clock1/1 -> Clutch 3/1(Input)
  Switch 1/1 -> Sine Wave 2/1, Sine Wave 4/1, Sine Wave 1/1, Sine Wave 3/1
  Constant 3/1 -> Switch 1/3
  Constant 4/1 -> Sum3/1
  Sum3/1 -> Switch 1/1
  Constant 5/1 -> Switch 2/1
  Switch 2/1 -> Product 4/2
  Mux12/1 -> Sum4/1
  Mux1/1 -> Sum4/2
  Constant 7/1 -> Product 4/1
  Constant 8/1 -> Switch 3/1
  Constant 6/1 -> Switch 3/3
  Constant 2/1 -> Switch 4/1
  Switch 4/1 -> Sum1/1
  Constant 1/1 -> Switch 4/3
  Switch 3/1 -> Mux1/1
  Constant 9/1 -> Switch 5/3
  Constant 10/1 -> Switch 5/1
  Product 4/1 -> Sum6/1
  Sum6/1 -> Mux1/2
  Switch 5/1 -> Sum6/2
  Sum4/1 -> X*/1
  Constant 12/1 -> Switch 6/1
  Constant 11/1 -> Switch 6/3
  Switch 6/1 -> Sum2/1
  Clutch 3/1(Output) -> Switch 6/2, Switch 2/2, Switch 5/2, Switch 3/2, Switch 2/3, Switch 1/2, Switch 4/2, Sum3/2

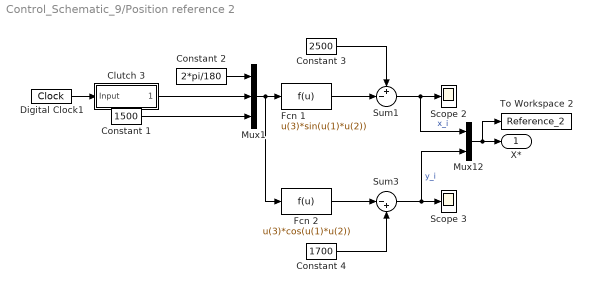
== system Control_Schematic_9/Position reference 2 ==
  Clutch 3 : Subsystem
  Constant 1 : Constant  Value=1500
  Constant 2 : Constant  Value=2*pi/180
  Constant 3 : Constant  Value=2500
  Constant 4 : Constant  Value=1700
  Digital Clock1 : DigitalClock  SampleTime=Ts
  Fcn 1 : Fcn  Expr=u(3)*sin(u(1)*u(2))
  Fcn 2 : Fcn  Expr=u(3)*cos(u(1)*u(2))
  Mux1 : Mux  Inputs=3
  Mux12 : Mux  Inputs=2
  Scope 2 : Scope
      settings: YMin=-10  YMax=10
  Scope 3 : Scope
      settings: YMin=-10  YMax=10
  Sum1 : Sum  Inputs=+-|
  Sum3 : Sum  Inputs=|-+
  To Workspace 2 : ToWorkspace  VariableName=Reference_2  SaveFormat=Structure With Time  SampleTime=-1
  X* : Outport
  wires:
  Constant 1/1 -> Mux1/3
  Digital Clock1/1 -> Clutch 3/1(Input)
  Sum1/1 -> Mux12/1, Scope 2/1  "x_i"
  Mux12/1 -> To Workspace 2/1, X*/1
  Clutch 3/1(Output) -> Mux1/2
  Constant 3/1 -> Sum1/1
  Constant 2/1 -> Mux1/1
  Constant 4/1 -> Sum3/2
  Sum3/1 -> Scope 3/1, Mux12/2  "y_i"
  Fcn 1/1 -> Sum1/2
  Mux1/1 -> Fcn 2/1, Fcn 1/1
  Fcn 2/1 -> Sum3/1

== system Control_Schematic_9/Position reference 3 ==
  Constant 3 : Constant  Value=1000
  Constant 4 : Constant  Value=4000
  Mux12 : Mux  Inputs=2
  To Workspace 2 : ToWorkspace  VariableName=Reference_3  SaveFormat=Structure With Time  SampleTime=-1
  X* : Outport
  wires:
  Mux12/1 -> X*/1, To Workspace 2/1
  Constant 4/1 -> Mux12/2
  Constant 3/1 -> Mux12/1

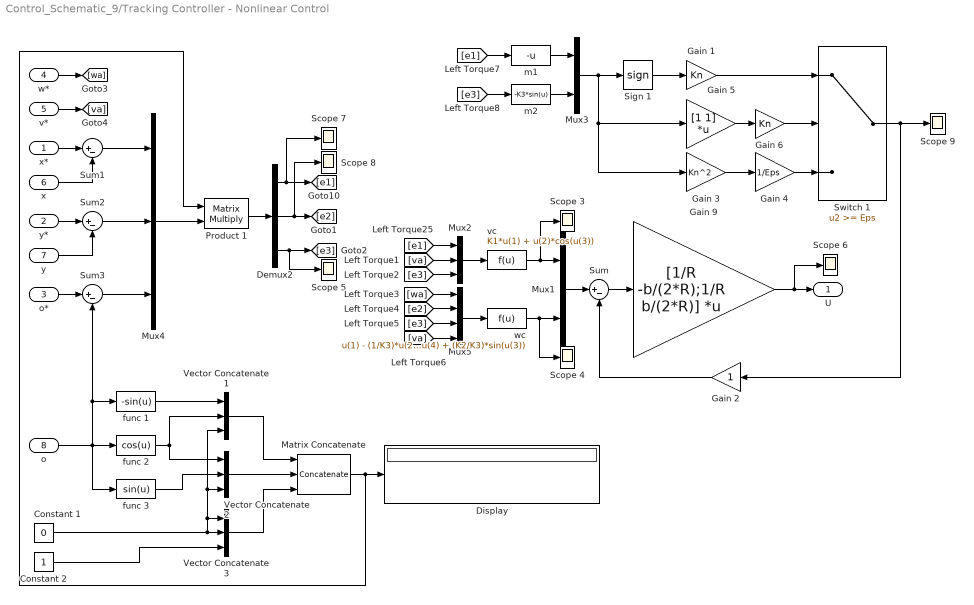
== system Control_Schematic_9/Tracking Controller - Nonlinear Control ==
  x* : Inport
  y* : Inport  Port=2
  o* : Inport  Port=3
  w* : Inport  Port=4
  v* : Inport  Port=5
  x : Inport  Port=6
  y : Inport  Port=7
  o : Inport  Port=8
  Constant 1 : Constant  Value=0
  Constant 2 : Constant
  Demux2 : Demux  Outputs=3
  Display : Display
  Gain 1 : Gain  Gain=Kn
  Gain 2 : Gain
  Gain 3 : Gain  Gain=Kn^2
  Gain 4 : Gain  Gain=1/Eps
  Gain 5 : Gain  Gain=[1 1]  Multiplication=Matrix(K*u)
  Gain 6 : Gain  Gain=Kn
  Gain 9 : Gain  Gain=[1/R -b/(2*R);1/R b/(2*R)]  Multiplication=Matrix(K*u)
  Matrix Concatenate : Concatenate  NumInputs=3  Mode=Multidimensional array  ConcatenateDimension=2
  Mux1 : Mux  Inputs=2
  Mux2 : Mux  Inputs=3
  Mux3 : Mux  Inputs=2
  Mux4 : Mux  Inputs=3
  Mux5 : Mux
  Product 1 : Product  Multiplication=Matrix(*)
  Scope {3..9} (7 alike) : Scope
      Scope 3 settings: YMin=-10  YMax=10  SaveName=ScopeData44
      Scope 4 settings: YMin=-400  YMax=1300  SaveName=ScopeData45
      Scope 5 settings: YMin=-8  YMax=-1.75  SaveName=ScopeData47
      Scope 6 settings: TimeRange=388.54  YMin=-0.5  YMax=0.5  SaveName=ScopeData12
      Scope 7 settings: YMin=-10  YMax=10  SaveName=ScopeData48
      Scope 8 settings: YMin=-10  YMax=10  SaveName=ScopeData49
      Scope 9 settings: YMin=-0.1  YMax=0.1  SaveName=ScopeData50
  Sign 1 : Signum
  Sum{,1..3} (4 alike) : Sum  Inputs=|+-
  Switch 1 : Switch  Threshold=Eps
  Vector Concatenate 1 : Concatenate  NumInputs=3
  Vector Concatenate 2 : Concatenate  NumInputs=3
  Vector Concatenate 3 : Concatenate  NumInputs=3
  func 1 : Fcn  Expr=-sin(u)
  func 2 : Fcn  Expr=cos(u)
  func 3 : Fcn  Expr=sin(u)
  m1 : Fcn  Expr=-u
  m2 : Fcn  Expr=-K3*sin(u)
  vc : Fcn  Expr=K1*u(1) + u(2)*cos(u(3))
  wc : Fcn  Expr=u(1) - (1/K3)*u(2)*u(4) + (K2/K3)*sin(u(3))
  U : Outport
  wires:
  Gain 9/1 -> Scope 6/1, U/1
  wc/1 -> Scope 4/1, Mux1/2
  vc/1 -> Scope 3/1, Mux1/1
  Sum/1 -> Gain 9/1
  m2/1 -> Mux3/2
  m1/1 -> Mux3/1
  Mux3/1 -> Gain 5/1, Gain 3/1, Sign 1/1
  Sign 1/1 -> Gain 1/1
  Mux1/1 -> Sum/1
  func 2/1 -> Vector Concatenate 1/2, Vector Concatenate 2/1
  func 3/1 -> Vector Concatenate 2/2
  func 1/1 -> Vector Concatenate 1/1
  o/1 -> func 3/1, func 2/1, Sum3/2, func 1/1
  Constant 1/1 -> Vector Concatenate 3/1, Vector Concatenate 2/3, Vector Concatenate 1/3, Vector Concatenate 3/2
  Constant 2/1 -> Vector Concatenate 3/3
  Matrix Concatenate/1 -> Product 1/1, Display/1
  Vector Concatenate 1/1 -> Matrix Concatenate/1
  Vector Concatenate 2/1 -> Matrix Concatenate/2
  Vector Concatenate 3/1 -> Matrix Concatenate/3
  x*/1 -> Sum1/1
  x/1 -> Sum1/2
  y*/1 -> Sum2/1
  y/1 -> Sum2/2
  o*/1 -> Sum3/1
  Sum3/1 -> Mux4/3
  Sum1/1 -> Mux4/1
  Sum2/1 -> Mux4/2
  Mux4/1 -> Product 1/2
  Product 1/1 -> Demux2/1
  Demux2/1 -> Scope 7/1, [e1]
  Demux2/2 -> Scope 8/1, [e2]
  Demux2/3 -> Scope 5/1, [e3]
  [e1] -> Mux2/1
  w*/1 -> [wa]
  v*/1 -> [va]
  [va] -> Mux2/2
  [e3] -> Mux2/3
  Mux2/1 -> vc/1
  Mux5/1 -> wc/1
  [wa] -> Mux5/1
  [e2] -> Mux5/2
  [e3] -> Mux5/3
  [va] -> Mux5/4
  [e1] -> m1/1
  [e3] -> m2/1
  Gain 2/1 -> Sum/2
  Gain 3/1 -> Gain 4/1
  Gain 5/1 -> Gain 6/1
  Gain 4/1 -> Switch 1/3
  Gain 6/1 -> Switch 1/2
  Gain 1/1 -> Switch 1/1
  Switch 1/1 -> Scope 9/1, Gain 2/1

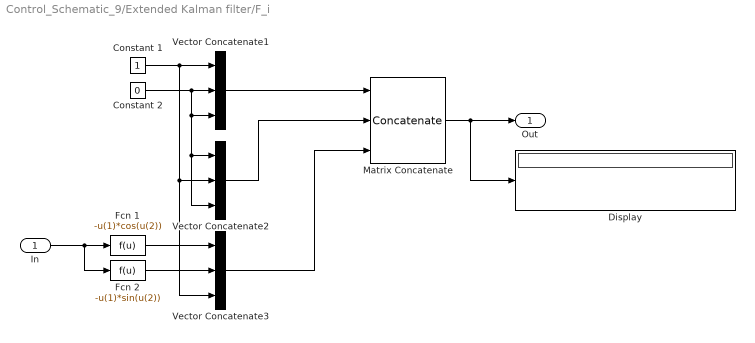
== system Control_Schematic_9/Extended Kalman filter/F_i ==
  In : Inport
  Constant 1 : Constant
  Constant 2 : Constant  Value=0
  Display : Display
  Fcn 1 : Fcn  Expr=-u(1)*cos(u(2))
  Fcn 2 : Fcn  Expr=-u(1)*sin(u(2))
  Matrix Concatenate : Concatenate  NumInputs=3  Mode=Multidimensional array  ConcatenateDimension=2
  Vector Concatenate1 : Concatenate  NumInputs=3
  Vector Concatenate2 : Concatenate  NumInputs=3
  Vector Concatenate3 : Concatenate  NumInputs=3
  Out : Outport
  wires:
  In/1 -> Fcn 2/1, Fcn 1/1
  Matrix Concatenate/1 -> Display/1, Out/1
  Constant 1/1 -> Vector Concatenate3/3, Vector Concatenate2/2, Vector Concatenate1/1
  Constant 2/1 -> Vector Concatenate2/3, Vector Concatenate2/1, Vector Concatenate1/3, Vector Concatenate1/2
  Vector Concatenate1/1 -> Matrix Concatenate/1
  Vector Concatenate2/1 -> Matrix Concatenate/2
  Fcn 1/1 -> Vector Concatenate3/1
  Fcn 2/1 -> Vector Concatenate3/2
  Vector Concatenate3/1 -> Matrix Concatenate/3

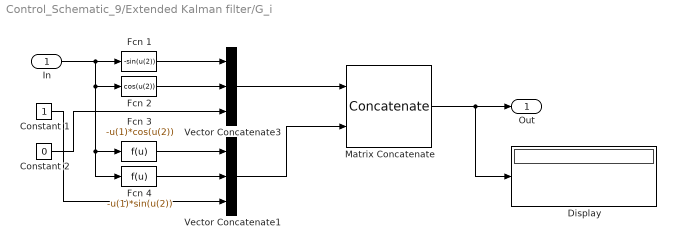
== system Control_Schematic_9/Extended Kalman filter/G_i ==
  In : Inport
  Constant 1 : Constant
  Constant 2 : Constant  Value=0
  Display : Display
  Fcn 1 : Fcn  Expr=-sin(u(2))
  Fcn 2 : Fcn  Expr=cos(u(2))
  Fcn 3 : Fcn  Expr=-u(1)*cos(u(2))
  Fcn 4 : Fcn  Expr=-u(1)*sin(u(2))
  Matrix Concatenate : Concatenate  Mode=Multidimensional array  ConcatenateDimension=2
  Vector Concatenate1 : Concatenate  NumInputs=3
  Vector Concatenate3 : Concatenate  NumInputs=3
  Out : Outport
  wires:
  Fcn 2/1 -> Vector Concatenate3/2
  Fcn 1/1 -> Vector Concatenate3/1
  Matrix Concatenate/1 -> Display/1, Out/1
  In/1 -> Fcn 1/1, Fcn 2/1, Fcn 4/1, Fcn 3/1
  Vector Concatenate3/1 -> Matrix Concatenate/1
  Vector Concatenate1/1 -> Matrix Concatenate/2
  Constant 2/1 -> Vector Concatenate3/3
  Constant 1/1 -> Vector Concatenate1/3
  Fcn 3/1 -> Vector Concatenate1/1
  Fcn 4/1 -> Vector Concatenate1/2

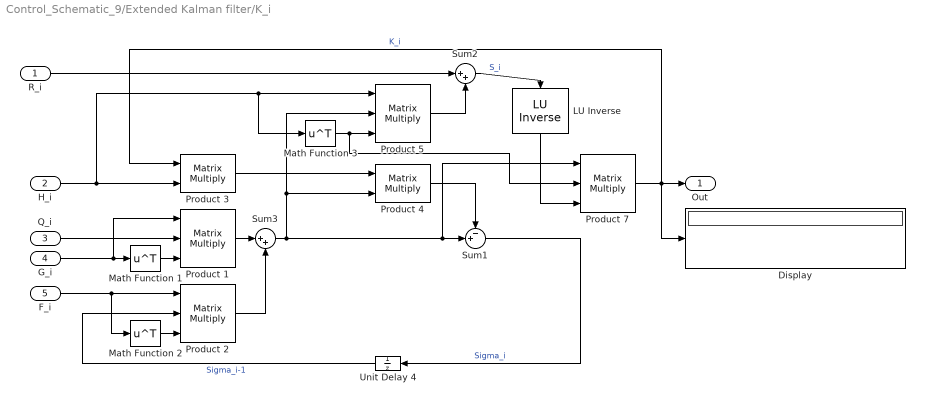
== system Control_Schematic_9/Extended Kalman filter/K_i ==
  R_i : Inport
  H_i : Inport  Port=2
  Q_i : Inport  Port=3
  G_i : Inport  Port=4
  F_i : Inport  Port=5
  " LU Inverse" : dspinverses/ LU Inverse
  Display : Display
  Math Function 1 : Math  Operator=transpose  SaturateOnIntegerOverflow=on
  Math Function 2 : Math  Operator=transpose  SaturateOnIntegerOverflow=on
  Math Function 3 : Math  Operator=transpose  SaturateOnIntegerOverflow=on
  Product {1..2,5,7} (4 alike) : Product  Inputs=3  Multiplication=Matrix(*)
  Product 3 : Product  Multiplication=Matrix(*)
  Product 4 : Product  Multiplication=Matrix(*)
  Sum1 : Sum  Inputs=-+|
  Sum2 : Sum  Inputs=|++
  Sum3 : Sum  Inputs=|++
  Unit Delay 4 : UnitDelay  InitialCondition=[1 0 0;0 1 0;0 0 1]  SampleTime=-1
  Out : Outport
  wires:
  Q_i/1 -> Product 1/2
  G_i/1 -> Math Function 1/1, Product 1/1
  Math Function 1/1 -> Product 1/3
  F_i/1 -> Math Function 2/1, Product 2/1
  Unit Delay 4/1 -> Product 2/2  "Sigma_i-1"
  Math Function 2/1 -> Product 2/3
  Product 1/1 -> Sum3/1
  Product 2/1 -> Sum3/2
  H_i/1 -> Product 5/1, Math Function 3/1, Product 3/2
  Product 7/1 -> Out/1, Display/1, Product 3/1  "K_i"
  Product 3/1 -> Product 4/1
  Sum3/1 -> Product 7/1, Sum1/2, Product 4/2, Product 5/2
  Product 4/1 -> Sum1/1
  Sum1/1 -> Unit Delay 4/1  "Sigma_i"
  Math Function 3/1 -> Product 5/3, Product 7/2
  R_i/1 -> Sum2/1
  Product 5/1 -> Sum2/2
  Sum2/1 -> " LU Inverse"/1  "S_i"
  " LU Inverse"/1 -> Product 7/3

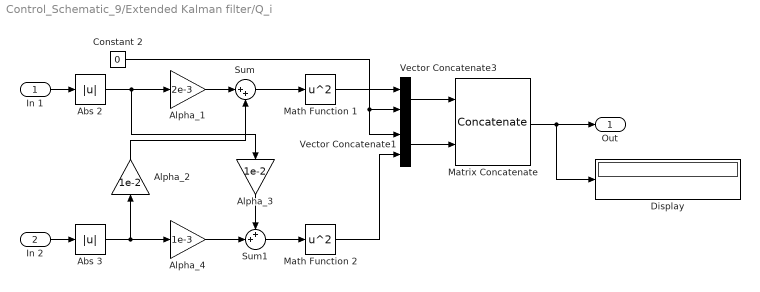
== system Control_Schematic_9/Extended Kalman filter/Q_i ==
  In 1 : Inport
  In 2 : Inport  Port=2
  Abs 2 : Abs
  Abs 3 : Abs
  Alpha_1 : Gain  Gain=2e-3
  Alpha_2 : Gain  Gain=1e-2
  Alpha_3 : Gain  Gain=1e-2
  Alpha_4 : Gain  Gain=1e-3
  Constant 2 : Constant  Value=0
  Display : Display
  Math Function 1 : Math  Operator=square  SaturateOnIntegerOverflow=on
  Math Function 2 : Math  Operator=square  SaturateOnIntegerOverflow=on
  Matrix Concatenate : Concatenate  Mode=Multidimensional array  ConcatenateDimension=2
  Sum : Sum  Inputs=|++
  Sum1 : Sum  Inputs=++|
  Vector Concatenate1 : Concatenate
  Vector Concatenate3 : Concatenate
  Out : Outport
  wires:
  Vector Concatenate1/1 -> Matrix Concatenate/2
  Vector Concatenate3/1 -> Matrix Concatenate/1
  Matrix Concatenate/1 -> Display/1, Out/1
  In 1/1 -> Abs 2/1
  In 2/1 -> Abs 3/1
  Abs 2/1 -> Alpha_3/1, Alpha_1/1
  Abs 3/1 -> Alpha_4/1, Alpha_2/1
  Constant 2/1 -> Vector Concatenate3/2, Vector Concatenate1/1
  Alpha_1/1 -> Sum/1
  Alpha_2/1 -> Sum/2
  Sum/1 -> Math Function 1/1
  Math Function 1/1 -> Vector Concatenate3/1
  Alpha_4/1 -> Sum1/2
  Alpha_3/1 -> Sum1/1
  Sum1/1 -> Math Function 2/1
  Math Function 2/1 -> Vector Concatenate1/2

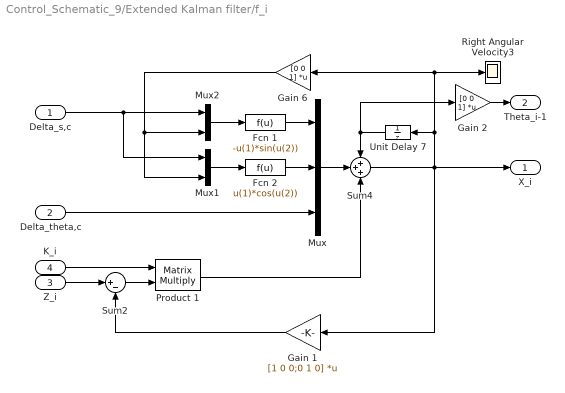
== system Control_Schematic_9/Extended Kalman filter/f_i ==
  Delta_s,c : Inport
  Delta_theta,c : Inport  Port=2
  Z_i : Inport  Port=3
  K_i : Inport  Port=4
  Fcn 1 : Fcn  Expr=-u(1)*sin(u(2))
  Fcn 2 : Fcn  Expr=u(1)*cos(u(2))
  Gain 1 : Gain  Gain=[1 0 0;0 1 0]  Multiplication=Matrix(K*u)
  Gain 2 : Gain  Gain=[0 0 1]  Multiplication=Matrix(K*u)
  Gain 6 : Gain  Gain=[0 0 1]  Multiplication=Matrix(K*u)
  Mux : Mux  Inputs=3
  Mux1 : Mux  Inputs=2
  Mux2 : Mux  Inputs=2
  Product 1 : Product  Multiplication=Matrix(*)
  Right Angular Velocity3 : Scope
      settings: YMin=-1  YMax=1  SaveName=ScopeData30
  Sum2 : Sum  Inputs=|+-
  Sum4 : Sum  Inputs=+++
  Unit Delay 7 : UnitDelay  InitialCondition=[2500 200 0]'  SampleTime=-1
  X_i : Outport
  Theta_i-1 : Outport  Port=2
  wires:
  Mux1/1 -> Fcn 2/1
  Delta_s,c/1 -> Mux1/1, Mux2/1
  Delta_theta,c/1 -> Mux/3
  Mux2/1 -> Fcn 1/1
  Fcn 1/1 -> Mux/1
  Fcn 2/1 -> Mux/2
  Sum4/1 -> X_i/1, Gain 1/1, Unit Delay 7/1, Right Angular Velocity3/1, Gain 6/1
  Gain 6/1 -> Mux1/2, Mux2/2
  Z_i/1 -> Sum2/1
  Gain 1/1 -> Sum2/2
  Sum2/1 -> Product 1/2
  K_i/1 -> Product 1/1
  Unit Delay 7/1 -> Gain 2/1, Sum4/1
  Mux/1 -> Sum4/2
  Product 1/1 -> Sum4/3
  Gain 2/1 -> Theta_i-1/1

== system Control_Schematic_9/Mobile robot/ADAMS Plant ==
  ADAMS inputs : Inport
  S-Function : S-Function  StopFcn=clear mex  FunctionName=adams_plant  Parameters=exevie,exesol,stat,outfil,nampre,o_rate,nam_in,namout,dft,modsim,modani,dt_out,inicmd,exetyp,comtyp,ada_host, workdir,pin_interp_order,pout_extrap_order,pin_extrap_order,pout_interp_order,simulink_lead_cosim  EnableBusSupport=off
  ADAMS outputs : Outport  InitialOutput=0
  wires:
  S-Function/1 -> ADAMS outputs/1
  ADAMS inputs/1 -> S-Function/1

== system Control_Schematic_9/Position reference 1/Clutch 3 ==
  Input : Inport
  Constant1 : Constant
  Digital Clock : DigitalClock  SampleTime=Ts
  Product : Product
  Rear Wheel Angular Speed5 : Scope
      settings: YMin=2.77556e-17  YMax=1  SaveName=ScopeData20
  Sine Wave : Sin  Frequency=(pi/40)  SampleTime=Ts
  Switch : Switch  Threshold=20
  Output : Outport
  wires:
  Constant1/1 -> Switch/1
  Digital Clock/1 -> Switch/2
  Switch/1 -> Rear Wheel Angular Speed5/1, Product/1
  Input/1 -> Product/2
  Product/1 -> Output/1
  Sine Wave/1 -> Switch/3

== system Control_Schematic_9/Position reference 2/Clutch 3 ==
  Input : Inport
  Constant1 : Constant
  Digital Clock : DigitalClock  SampleTime=Ts
  Product : Product
  Rear Wheel Angular Speed5 : Scope
      settings: YMin=2.77556e-17  YMax=1  SaveName=ScopeData20
  Sine Wave : Sin  Frequency=(pi/40)  SampleTime=Ts
  Switch : Switch  Threshold=20
  Output : Outport
  wires:
  Constant1/1 -> Switch/1
  Digital Clock/1 -> Switch/2
  Switch/1 -> Rear Wheel Angular Speed5/1, Product/1
  Input/1 -> Product/2
  Product/1 -> Output/1
  Sine Wave/1 -> Switch/3
